simulink model "Response"  (R2019a)
settings: Solver=VariableStepAuto  StartTime=0.0  StopTime=20  FixedStep=1  RelTol=1e-3
settings Model: Creator=omare  LastModifiedBy=omare

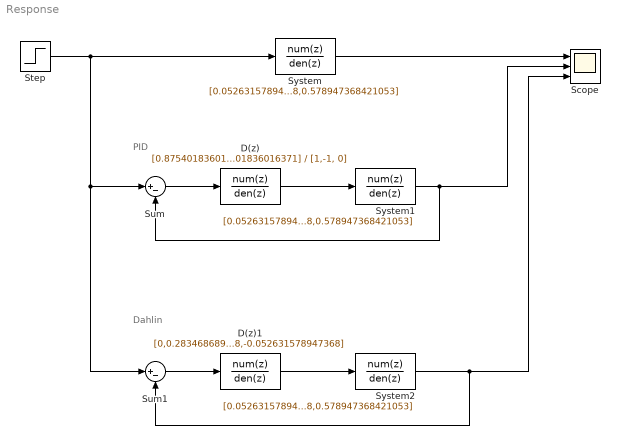
== system Response ==
  note: Dahlin
  note: PID
  D(z) : DiscreteTransferFcn  Numerator=[0.875401836016371,1.750803672032744,0.875401836016371]  Denominator=[1,-1, 0]  SampleTime=1
  D(z)1 : DiscreteTransferFcn  Numerator=[0,0.283468689426211,0.208871665892997,0.164113451773069]  Denominator=[0.052631578947368,0.052631578947368,-0.052631578947368,-0.052631578947368]  SampleTime=1
  Scope : Scope  NumInputPorts=3
  Step : Step  After=3  SampleTime=1
  Sum : Sum  Inputs=|+-
  Sum1 : Sum  Inputs=|+-
  System : DiscreteTransferFcn  Numerator=[0.052631578947368,0.105263157894737,0.052631578947368]  Denominator=[1,0.736842105263158,0.578947368421053]  SampleTime=1
  System1 : DiscreteTransferFcn  Numerator=[0.052631578947368,0.105263157894737,0.052631578947368]  Denominator=[1,0.736842105263158,0.578947368421053]  SampleTime=1
  System2 : DiscreteTransferFcn  Numerator=[0.052631578947368,0.105263157894737,0.052631578947368]  Denominator=[1,0.736842105263158,0.578947368421053]  SampleTime=1
  wires:
  System/1 -> Scope/1
  System1/1 -> Scope/2, Sum/2
  System2/1 -> Scope/3, Sum1/2
  Sum/1 -> D(z)/1
  D(z)/1 -> System1/1
  Step/1 -> Sum1/1, Sum/1, System/1
  Sum1/1 -> D(z)1/1
  D(z)1/1 -> System2/1
